simulink model "lab2_1_simulink"  (R2023a)
settings: Solver=FixedStepAuto  StartTime=0.0  StopTime=10.0  FixedStep=0.01  MaxStep=0.001  MinStep=0.001  RelTol=1e-3
settings Model: Creator=george theologis  LastModifiedBy=george theologis
settings SolverCC: InitialStep=0.001

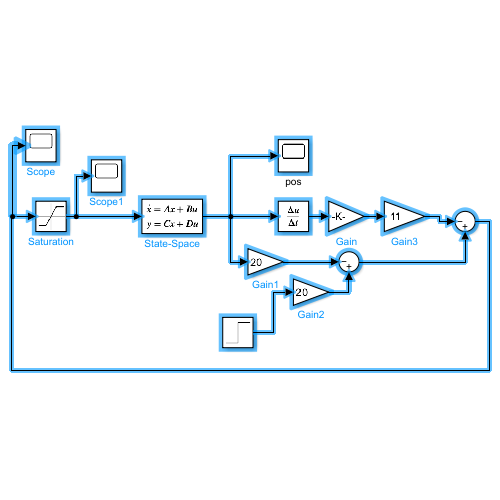
[thumbnail: Simulink's stored preview of the top-level diagram]
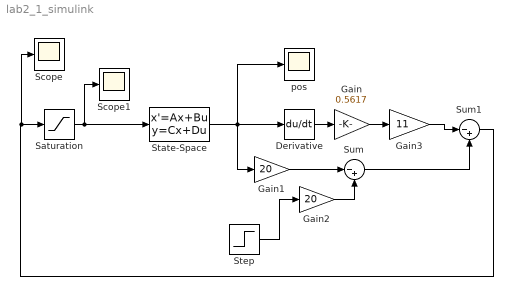
== system lab2_1_simulink ==
  Derivative : Derivative
  Gain : Gain  Gain=0.5617
  Gain1 : Gain  Gain=20
  Gain2 : Gain  Gain=20
  Gain3 : Gain  Gain=11
  Saturation : Saturate  UpperLimit=10  LowerLimit=-10
  Scope : Scope
  Scope1 : Scope
  State-Space : StateSpace  A=|  B=[0;1.6906;]  C=[1 0]  D=0  InitialCondition=[2;0;]
      | [0 1.7802
      | ;0 1/0.53;]
  Step : Step  Time=0  After=5  SampleTime=0
  Sum : Sum  Inputs=|-+
  Sum1 : Sum  Inputs=|-+
  pos : Scope
  wires:
  State-Space/1 -> Derivative/1, Gain1/1, pos/1
  Gain1/1 -> Sum/1
  Step/1 -> Gain2/1
  Gain2/1 -> Sum/2
  Gain/1 -> Gain3/1
  Gain3/1 -> Sum1/1
  Sum/1 -> Sum1/2
  Derivative/1 -> Gain/1
  Sum1/1 -> Scope/1, Saturation/1
  Saturation/1 -> State-Space/1, Scope1/1
